simulink model "ON"  (R2025b)
settings: Solver=VariableStepAuto  StartTime=0.0  StopTime=300  FixedStep=0.5  RelTol=1e-3
InitFcn:
  | mdlWks = get_param(gcs,'ModelWorkspace');
  | a = getVariable(mdlWks,'a');
  | b = getVariable(mdlWks,'b');
  | c = getVariable(mdlWks,'c');
StopFcn:
  | fTraj = findobj("Tag","asbAUVTrajectory");
  | 
  | if isempty(fTraj)
  |    fTraj = figure("Tag","asbAUVTrajectory");
  |    axes(fTraj);
  | end
  | 
  | axTraj= gca(fTraj);
  | 
  | if exist('PositionData', 'var')
  |    plot3(axTraj,PositionData(1,1),PositionData(1,2),PositionData(1,3),'r*')
  |    hold on
  |    plot3(axTraj,PositionData(:,1),PositionData(:,2),PositionData(:,3));
  |    plot3(axTraj,PositionData(end,1),PositionData(end,2),PositionData(end,3),'g*');
  | 
  |    axTraj.XLim = [0 15];
  |    axTraj.YLim = [-10 2];
  |    axTraj.ZLim = [-2 12];
  |    axTraj.XLabel.String = 'X (m)';
  |    axTraj.YLabel.String = 'Y (m)';
  |    axTraj.ZLabel.String = 'Z (m)';
  |    grid on
  |    hold off
  | 
  |    legend(axTraj,{'Start Point','Trajectory','End Point'});
  | end
model workspace (MAT data in the model file):
  a = 1
  b = 0
  c = 1
libraries: asbAUVlib x28, dspfdesign x6, slpidlib x6, aerolibobsolete x1, aerolibasang x1, sharedutil x1, aerolibnav x1, SignalEditorBlockLib x1
(part 1 of 3)
CloseFcn:
  | fTraj = findobj("Tag","asbAUVTrajectory");
  | fFig = findobj("Tag","asbAUVFigure");
  | 
  | if ~isempty(fTraj)
  |    close(fTraj);
  | end
  | if ~isempty(fFig)
  |    close(fFig);
  | end
  | 
  | % clean up base workspace variables from InitFcn
  | clear a b c mdlWks;
  | % clean up base workspace variables from figure window
  | clear fTraj fFig axTraj;
settings Model: Creator=The MathWorks, Inc.  LastModifiedBy=luke
settings SolverCC: AlgebraicLoopSolver=TrustRegion
settings DataIOCC: ReturnWorkspaceOutputs=off
settings OptimizationCC: ReuseModelBlockBuffer=off
settings DebuggingCC: UnconnectedInputMsg=warning  UnconnectedOutputMsg=warning  UnconnectedLineMsg=warning  ArithmeticOperatorsInVariantConditions=warning
settings ModelReferenceCC: EnableRefExpFcnMdlSchedulingChecks=on
settings SFSimCC: CustomCodeUndefinedFunction=UseInterfaceOnly
settings RTWCC: GPUComputeCapability=3.5  DLArmComputeVersion=19.05

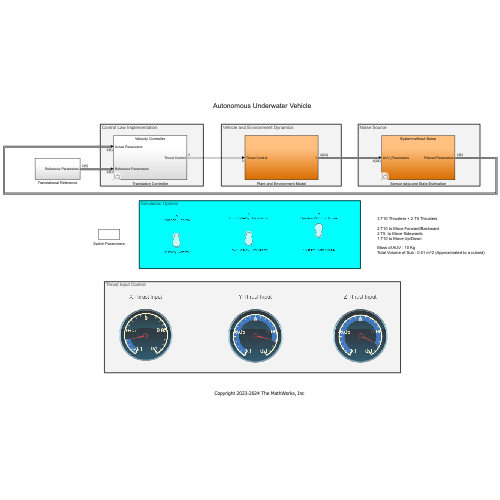
[thumbnail: Simulink's stored preview of the top-level diagram]
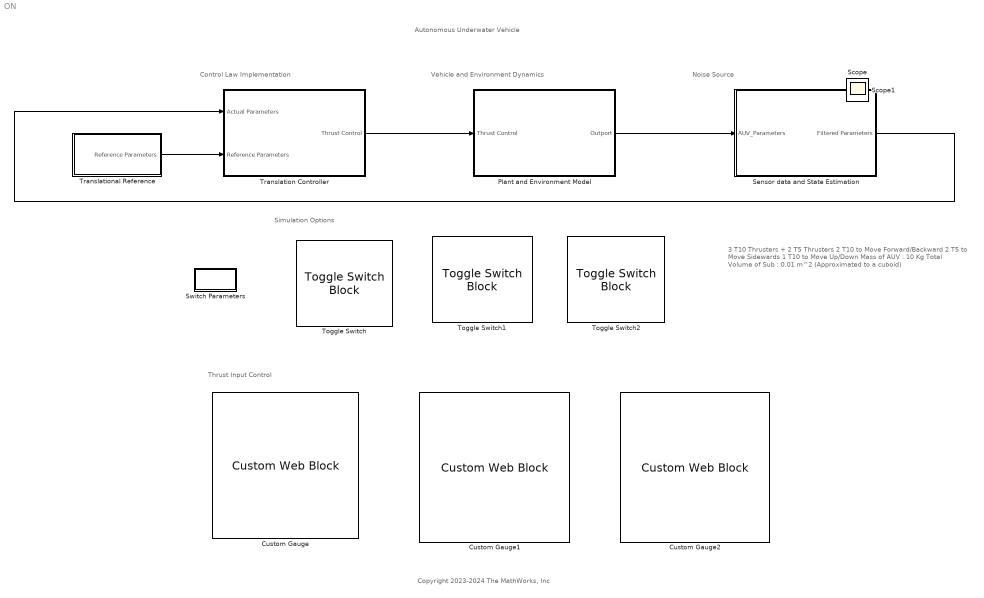
== system ON ==
  note: Thrust Input Control
  note: Control Law Implementation
  note: Noise Source
  note: Vehicle and Environment Dynamics
  note: Simulation Options
  note: Autonomous Underwater Vehicle
  note: 3 T10 Thrusters + 2 T5 Thrusters
      |
      | 2 T10 to Move Forward/Backward
      | 2 T5 to Move Sidewards
      | 1 T10 to Move Up/Down
      |
      | Mass of AUV : 10 Kg
      | Total Volume of Sub : 0.01 m^2 (Approximated to a cuboid)
  note: Copyright 2023-2024 The MathWorks, Inc
  Custom Gauge : CustomWebBlock  ShowInitialText=on  Configuration="{\"components\":[{\"name\":\"CircularScaleComponent\",\"settings\":{\"bounds\":{\"max\":0.1,\"min\":-0.1,\"tickInterval\":\"auto\"},\"direction\":\"cw\",\"flipLimits\":0,\"innerRadius\":0.5172763687199098,\"internalTickHeightScaleFactor\":1,\"labelColor\":[250,245,200],\"labelFont\":{\"font\":\"Arial\",\"fontSize\":12},\"labelRadius\":0.528,\"labelTransparency\":1,\"labelTrasparency\":1,\"minorTickHeightScaleFactor\":0.2,\"needleImage\":{\"size\":[200,50],\"src\":\"data:image\\/svg+xml;base64,PD94bWwgdmVyc2lvbj0iMS4wIiBlbmNvZGluZz0idXRmLTgiPz4KPCEtLSBHZW5lcmF0b3I6IEFkb2JlIElsbHVzdHJhdG9yIDE5LjIuMSwgU1ZHIEV4cG9ydCBQbHVnLUluIC4gU1ZHIFZlcnNpb246IDYuMDAgQnVpbGQgMCkgIC0tPgo8c3ZnIHZlcnNpb249IjEuMSIgeG1sbnM9Imh0dHA6Ly93d3cudzMub3JnLzIwMDAvc3ZnIiB4bWxuczp4bGluaz0iaHR0cDovL3d3dy53My5vcmcvMTk5OS94bGluayIgeD0iMHB4IiB5PSIwcHgiCgkgdmlld0JveD0iMCAwIDIwMCA1MCIgc3R5bGU9ImVuYWJsZS1iYWNrZ3JvdW5kOm5ldyAw ...(+9940 chars)\"},\"needleOffset\":[0.0902465113423366,0],\"needleOrientation\":-45,\"needleRotation\":-180,\"needleSize\":{\"height\":0.09363426638196895,\"width\":0.3745370655278758},\"outerRadius\":0.6944548624524601,\"position\":[0.06486742424242424,0.05627705627705628,0.8917748917748918,0.8787878787878788],\"referencePoint\":\"auto\",\"scaleAngle\":299.999999999988,\"scaleAngleOffset\":119.46147497096791,\"scaleColors\":[],\"scaleColorsSize\":0.2,\"scaleDirection\":\"CW\",\"scalePosition\":[0,0,1,1],\"showLabels\":1,\"showMinorTicks\":1,\"showSpanLine\":1,\"showTicks\":1,\"tickColor\":[250,245,200],\"tickTransparency\":1,\"valueBarColor\":[23,89,176],\"valueBarPosition\":[0,0,1,1],\"valueBarSize\":0.2,\"valueBarTransparency\":1}},{\"name\":\"BackgroundImageComponent\",\"settings\":{\"image\":{\"size\":[500,500],\"src\":\"data:image\\/svg+xml;base64,PD94bWwgdmVyc2lvbj0iMS4wIiBlbmNvZGluZz0iVVRGLTgiIHN0YW5kYWxvbmU9Im5vIj8+CjwhLS0gR2VuZXJhdG9yOiBBZG9iZSBJbGx1c3RyYXRvciAxOS4yLjEsIFNWRyBFeHBvcnQgUGx1Zy1JbiAuIFNWRyBWZXJzaW9uOiA2LjAwIEJ1aWxkIDApICAtLT4KCjxzdmcKICAgeG1sbnM6ZGM9Imh0dHA6Ly9wdXJsLm9yZy9kYy9lbGVtZW50cy8xLjEvIgogICB4bWxuczpjYz0iaHR0cDovL2NyZWF0aXZlY29tbW9ucy5vcmcvbnMjIgogICB4bWxuczpyZGY9Imh0dHA6Ly93d3cudzMub3JnLzE5OTkvMDIvMjItcmRmLXN5bnRh ...(+9660 chars)\",\"srcOrientation\":\"horizontal\"},\"position\":[0,0,1,1],\"scaleMode\":\"0\"}},{\"name\":\"ForegroundImageComponent\",\"settings\":{\"image\":{\"size\":[0,0],\"src\":\"default\",\"srcOrientation\":[]},\"isForeground\":1,\"position\":[0,0,1,1],\"scaleMode\":\"0\"}}],\"derived\":{\"blockParameters\":{\"ForegroundColor\":[0.9803921568627451,0.9607843137254902,0.7843137254901961],\"Limits\":{\"Max\":0.1,\"Min\":-0.1,\"Ticks\":\"auto\"},\"ScaleColors\":[],\"ScaleDirection\":\"Clockwise\",\"ScaleMax\":0.1,\"ScaleMin\":-0.1,\"TickInterval\":\"auto\",\"fixedAspectRatio\":\"on\"}},\"settings\":{\"BindingType\":\"signal\",\"aspectRatio\":1,\"backgroundOffset\":0.14,\"fixedAspectRatio\":\"on\",\"orientation\":\"horizontal\",\"version\":\"R2023a\"},\"type\":\"CircularGauge\"}"
  Custom Gauge1 : CustomWebBlock  ShowInitialText=on  Configuration="{\"components\":[{\"name\":\"CircularScaleComponent\",\"settings\":{\"bounds\":{\"max\":0.1,\"min\":-0.1,\"tickInterval\":\"auto\"},\"direction\":\"cw\",\"flipLimits\":0,\"innerRadius\":0.511012744107412,\"internalTickHeightScaleFactor\":1,\"labelColor\":[250,245,200],\"labelFont\":{\"font\":\"Arial\",\"fontSize\":12},\"labelRadius\":0.528,\"labelTransparency\":1,\"labelTrasparency\":1,\"minorTickHeightScaleFactor\":0.2,\"needleImage\":{\"size\":[200,50],\"src\":\"data:image\\/svg+xml;base64,PD94bWwgdmVyc2lvbj0iMS4wIiBlbmNvZGluZz0idXRmLTgiPz4KPCEtLSBHZW5lcmF0b3I6IEFkb2JlIElsbHVzdHJhdG9yIDE5LjIuMSwgU1ZHIEV4cG9ydCBQbHVnLUluIC4gU1ZHIFZlcnNpb246IDYuMDAgQnVpbGQgMCkgIC0tPgo8c3ZnIHZlcnNpb249IjEuMSIgeG1sbnM9Imh0dHA6Ly93d3cudzMub3JnLzIwMDAvc3ZnIiB4bWxuczp4bGluaz0iaHR0cDovL3d3dy53My5vcmcvMTk5OS94bGluayIgeD0iMHB4IiB5PSIwcHgiCgkgdmlld0JveD0iMCAwIDIwMCA1MCIgc3R5bGU9ImVuYWJsZS1iYWNrZ3JvdW5kOm5ldyAw ...(+9940 chars)\"},\"needleOffset\":[0.0891537294102432,0],\"needleOrientation\":-45,\"needleRotation\":-180,\"needleSize\":{\"height\":0.09250046261487502,\"width\":0.37000185045950007},\"outerRadius\":0.6860458091266908,\"position\":[0.06486742424242424,0.05627705627705628,0.8917748917748918,0.8787878787878788],\"referencePoint\":\"auto\",\"scaleAngle\":299.999999999988,\"scaleAngleOffset\":119.46147497096791,\"scaleColors\":[],\"scaleColorsSize\":0.2,\"scaleDirection\":\"CW\",\"scalePosition\":[0,0,1,1],\"showLabels\":1,\"showMinorTicks\":1,\"showSpanLine\":1,\"showTicks\":1,\"tickColor\":[250,245,200],\"tickTransparency\":1,\"valueBarColor\":[23,89,176],\"valueBarPosition\":[0,0,1,1],\"valueBarSize\":0.2,\"valueBarTransparency\":1}},{\"name\":\"BackgroundImageComponent\",\"settings\":{\"image\":{\"size\":[500,500],\"src\":\"data:image\\/svg+xml;base64,PD94bWwgdmVyc2lvbj0iMS4wIiBlbmNvZGluZz0iVVRGLTgiIHN0YW5kYWxvbmU9Im5vIj8+CjwhLS0gR2VuZXJhdG9yOiBBZG9iZSBJbGx1c3RyYXRvciAxOS4yLjEsIFNWRyBFeHBvcnQgUGx1Zy1JbiAuIFNWRyBWZXJzaW9uOiA2LjAwIEJ1aWxkIDApICAtLT4KCjxzdmcKICAgeG1sbnM6ZGM9Imh0dHA6Ly9wdXJsLm9yZy9kYy9lbGVtZW50cy8xLjEvIgogICB4bWxuczpjYz0iaHR0cDovL2NyZWF0aXZlY29tbW9ucy5vcmcvbnMjIgogICB4bWxuczpyZGY9Imh0dHA6Ly93d3cudzMub3JnLzE5OTkvMDIvMjItcmRmLXN5bnRh ...(+9660 chars)\",\"srcOrientation\":\"horizontal\"},\"position\":[0,0,1,1],\"scaleMode\":\"0\"}},{\"name\":\"ForegroundImageComponent\",\"settings\":{\"image\":{\"size\":[0,0],\"src\":\"default\",\"srcOrientation\":[]},\"isForeground\":1,\"position\":[0,0,1,1],\"scaleMode\":\"0\"}}],\"derived\":{\"blockParameters\":{\"ForegroundColor\":[0.9803921568627451,0.9607843137254902,0.7843137254901961],\"Limits\":{\"Max\":0.1,\"Min\":-0.1,\"Ticks\":\"auto\"},\"ScaleColors\":[],\"ScaleDirection\":\"Clockwise\",\"ScaleMax\":0.1,\"ScaleMin\":-0.1,\"TickInterval\":\"auto\",\"fixedAspectRatio\":\"on\"}},\"settings\":{\"BindingType\":\"signal\",\"aspectRatio\":1,\"backgroundOffset\":0.14,\"fixedAspectRatio\":\"on\",\"orientation\":\"horizontal\",\"version\":\"R2023a\"},\"type\":\"CircularGauge\"}"
  Custom Gauge2 : CustomWebBlock  ShowInitialText=on  Configuration="{\"components\":[{\"name\":\"CircularScaleComponent\",\"settings\":{\"bounds\":{\"max\":0.1,\"min\":-0.1,\"tickInterval\":\"auto\"},\"direction\":\"cw\",\"flipLimits\":0,\"innerRadius\":0.4979572745541241,\"internalTickHeightScaleFactor\":1,\"labelColor\":[250,245,200],\"labelFont\":{\"font\":\"Arial\",\"fontSize\":12},\"labelRadius\":0.528,\"labelTransparency\":1,\"labelTrasparency\":1,\"minorTickHeightScaleFactor\":0.2,\"needleImage\":{\"size\":[200,50],\"src\":\"data:image\\/svg+xml;base64,PD94bWwgdmVyc2lvbj0iMS4wIiBlbmNvZGluZz0idXRmLTgiPz4KPCEtLSBHZW5lcmF0b3I6IEFkb2JlIElsbHVzdHJhdG9yIDE5LjIuMSwgU1ZHIEV4cG9ydCBQbHVnLUluIC4gU1ZHIFZlcnNpb246IDYuMDAgQnVpbGQgMCkgIC0tPgo8c3ZnIHZlcnNpb249IjEuMSIgeG1sbnM9Imh0dHA6Ly93d3cudzMub3JnLzIwMDAvc3ZnIiB4bWxuczp4bGluaz0iaHR0cDovL3d3dy53My5vcmcvMTk5OS94bGluayIgeD0iMHB4IiB5PSIwcHgiCgkgdmlld0JveD0iMCAwIDIwMCA1MCIgc3R5bGU9ImVuYWJsZS1iYWNrZ3JvdW5kOm5ldyAw ...(+9940 chars)\"},\"needleOffset\":[0.08687600969914216,0],\"needleOrientation\":-45,\"needleRotation\":-180,\"needleSize\":{\"height\":0.09013723980436975,\"width\":0.360548959217479},\"outerRadius\":0.6685185551071089,\"position\":[0.06486742424242424,0.05627705627705628,0.8917748917748918,0.8787878787878788],\"referencePoint\":\"auto\",\"scaleAngle\":299.999999999988,\"scaleAngleOffset\":119.46147497096791,\"scaleColors\":[],\"scaleColorsSize\":0.2,\"scaleDirection\":\"CW\",\"scalePosition\":[0,0,1,1],\"showLabels\":1,\"showMinorTicks\":1,\"showSpanLine\":1,\"showTicks\":1,\"tickColor\":[250,245,200],\"tickTransparency\":1,\"valueBarColor\":[23,89,176],\"valueBarPosition\":[0,0,1,1],\"valueBarSize\":0.2,\"valueBarTransparency\":1}},{\"name\":\"BackgroundImageComponent\",\"settings\":{\"image\":{\"size\":[500,500],\"src\":\"data:image\\/svg+xml;base64,PD94bWwgdmVyc2lvbj0iMS4wIiBlbmNvZGluZz0iVVRGLTgiIHN0YW5kYWxvbmU9Im5vIj8+CjwhLS0gR2VuZXJhdG9yOiBBZG9iZSBJbGx1c3RyYXRvciAxOS4yLjEsIFNWRyBFeHBvcnQgUGx1Zy1JbiAuIFNWRyBWZXJzaW9uOiA2LjAwIEJ1aWxkIDApICAtLT4KCjxzdmcKICAgeG1sbnM6ZGM9Imh0dHA6Ly9wdXJsLm9yZy9kYy9lbGVtZW50cy8xLjEvIgogICB4bWxuczpjYz0iaHR0cDovL2NyZWF0aXZlY29tbW9ucy5vcmcvbnMjIgogICB4bWxuczpyZGY9Imh0dHA6Ly93d3cudzMub3JnLzE5OTkvMDIvMjItcmRmLXN5bnRh ...(+9660 chars)\",\"srcOrientation\":\"horizontal\"},\"position\":[0,0,1,1],\"scaleMode\":\"0\"}},{\"name\":\"ForegroundImageComponent\",\"settings\":{\"image\":{\"size\":[0,0],\"src\":\"default\",\"srcOrientation\":[]},\"isForeground\":1,\"position\":[0,0,1,1],\"scaleMode\":\"0\"}}],\"derived\":{\"blockParameters\":{\"ForegroundColor\":[0.9803921568627451,0.9607843137254902,0.7843137254901961],\"Limits\":{\"Max\":0.1,\"Min\":-0.1,\"Ticks\":\"auto\"},\"ScaleColors\":[],\"ScaleDirection\":\"Clockwise\",\"ScaleMax\":0.1,\"ScaleMin\":-0.1,\"TickInterval\":\"auto\",\"fixedAspectRatio\":\"on\"}},\"settings\":{\"BindingType\":\"signal\",\"aspectRatio\":1,\"backgroundOffset\":0.14,\"fixedAspectRatio\":\"on\",\"orientation\":\"horizontal\",\"version\":\"R2023a\"},\"type\":\"CircularGauge\"}"
  Plant and Environment Model : Subsystem
  Sensor data and State Estimation : Subsystem  Variant=on
  Switch Parameters : Subsystem
      mask Display: text(0.5, 0.5, 'Switch Parameters', 'horizontalAlignment', 'center')
  Toggle Switch : ToggleSwitchBlock
  Toggle Switch1 : ToggleSwitchBlock
  Toggle Switch2 : ToggleSwitchBlock
  Translation Controller : Subsystem  Variant=on
  Translational Reference : Subsystem
  Scope : Scope
      settings: ActiveDisplayYMinimum=-10363.49442  ActiveDisplayYMaximum=1151.49938  DataLoggingVariableName=ScopeData2
  Scope1 : Scope
      settings: ActiveDisplayYMinimum=-1  ActiveDisplayYMaximum=1
  wires:
  Translational Reference/1(Reference Parameters) -> Translation Controller/2(Reference Parameters)
  Translation Controller/1(Thrust Control) -> Plant and Environment Model/1(Thrust Control)
  Plant and Environment Model/1(Outport) -> Sensor data and State Estimation/1(AUV_Parameters)
  Sensor data and State Estimation/1(Filtered Parameters) -> Translation Controller/1(Actual Parameters)
